simulink model "stellaris_lp_gmeter"  (R2017a)
settings: Solver=FixedStepDiscrete  StartTime=0.0  StopTime=10.0  FixedStep=0.01  RelTol=1e-3  EnableMultiTasking=on
undefined symbols (not defined in the file): C, T
libraries: stellaris_lp_lib x4
settings Model: ExtModeTrigDuration=2  Creator=peselnikmg  LastModifiedBy=Nilim
settings DataIOCC: LimitDataPoints=on  SaveFormat=Array  SignalLoggingSaveFormat=ModelDataLogs  ReturnWorkspaceOutputs=on
settings OptimizationCC: UseDivisionForNetSlopeComputation=on  UseFloatMulNetSlope=on  UseSpecifiedMinMax=on  PassReuseOutputArgsAs=Individual arguments  ExpressionDepthLimit=2147483647  ZeroExternalMemoryAtStartup=off  ZeroInternalMemoryAtStartup=off  NoFixptDivByZeroProtection=on  EfficientFloat2IntCast=on  LifeSpan=inf  MaxStackSize=64  OptimizeBlockOrder=speed
settings DebuggingCC: ReadBeforeWriteMsg=DisableAll  WriteAfterWriteMsg=DisableAll  WriteAfterReadMsg=DisableAll  MultiTaskDSMMsg=none  IntegerOverflowMsg=error  ParameterTunabilityLossMsg=error  AssertControl=DisableAll  StateNameClashWarn=warning  NonBusSignalsTreatedAsBus=error  SFInvalidInputDataAccessInChartInitDiag=error  SFTransitionOutsideNaturalParentDiag=error  SFUnreachableExecutionPathDiag=error  SFUndirectedBroadcastEventsDiag=error  SFExecutionAtInitializationDiag=none  IntegerSaturationMsg=error
settings HardwareCC: ProdBitPerPointer=32  ProdBitPerSizeT=32  ProdBitPerPtrDiffT=32  ProdLargestAtomicInteger=Long  ProdLargestAtomicFloat=Double  ProdWordSize=32  ProdHWDeviceType=ARM Compatible->ARM Cortex
settings ModelReferenceCC: UpdateModelReferenceTargets=IfOutOfDate  PropagateSignalLabelsOutOfModel=off
settings SFSimCC: SFSimEcho=off  MATLABDynamicMemAlloc=off
settings RTWCC: SystemTargetFile=ert.tlc  HardwareBoard=Tiva TM4C123G Launchpad  TLCOptions=-aInlineSetEventsForThisBaseRateFcn=TLC_FALSE -aSuppressMultiTaskScheduler=TLC_FALSE -aRateBasedStepFcn=1  TemplateMakefile=ert_default_tmf  Description=Embedded Coder  GenerateReport=on  RTWVerbose=off  Toolchain=Texas Instruments Code Composer Studio v6 (Tiva)  BuildConfiguration=Faster Runs  IncludeHyperlinkInReport=on  LaunchReport=on  GenerateTraceInfo=on  GenerateTraceReport=on  GenerateTraceReportSl=on  GenerateTraceReportSf=on  GenerateTraceReportEml=on
settings CodeAppCC: ForceParamTrailComments=on  IgnoreCustomStorageClasses=off  OperatorAnnotations=on  SimulinkDataObjDesc=on  SFDataObjDesc=on  MATLABFcnDesc=on  CustomSymbolStrType=$N$R$M  InsertBlockDesc=on  MATLABSourceComments=on  EnableCustomComments=on  ReqsInCode=on
settings ERTTargetCC: UtilityFuncGeneration=Shared location  CombineSignalStateStructs=on  SuppressErrorStatus=on  SupportNonFinite=off  ParenthesesLevel=Maximum  CastingMode=Standards  EnableSignedLeftShifts=off  EnableSignedRightShifts=off
settings ConfigComp: CovMetricSettings=dw  CovHtmlReporting=on  CovSaveCumulativeToWorkspaceVar=on  CovSaveSingleToWorkspaceVar=on  CovExternalEMLEnable=off

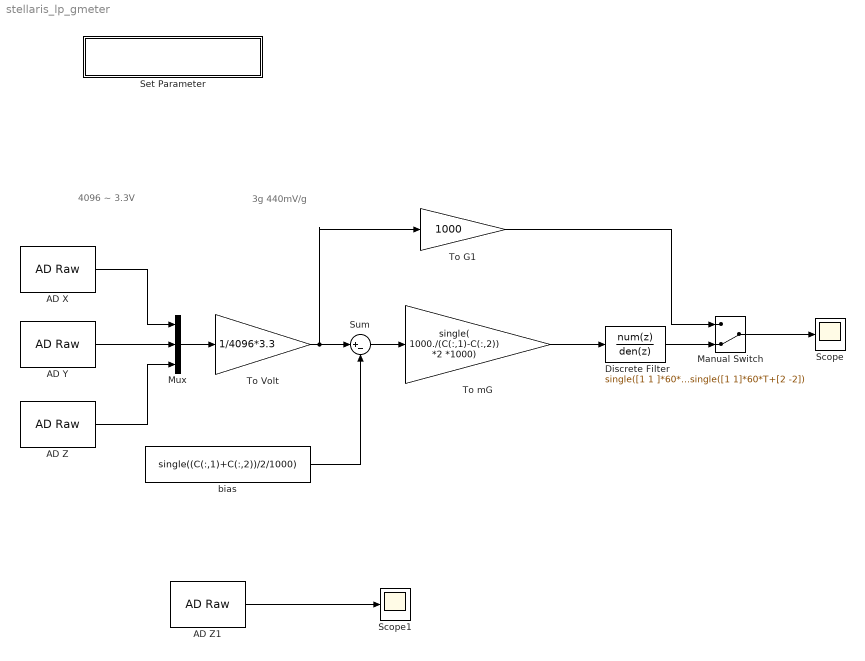
== system stellaris_lp_gmeter ==
  note: 4096 ~ 3.3V
  note: 3g 440mV/g
  AD X : stellaris_lp_lib/ADC/AD Raw  ch="1   PE3"  sample_time=0.01
      settings: SourceProductName=Run on Stellaris LaunchPad
  AD Y : stellaris_lp_lib/ADC/AD Raw  ch="2   PE2"  sample_time=0.01
      settings: SourceProductName=Run on Stellaris LaunchPad
  AD Z : stellaris_lp_lib/ADC/AD Raw  ch="3   PE1"  sample_time=0.01
      settings: SourceProductName=Run on Stellaris LaunchPad
  AD Z1 : stellaris_lp_lib/ADC/AD Raw  ch="4   PE0"  sample_time=0.02
      settings: SourceProductName=Run on Stellaris LaunchPad
  Discrete Filter : DiscreteFilter  Numerator=single([1 1 ]*60*T)  Denominator=single([1 1]*60*T+[2 -2])  InitialStates=single([0;0;0])
  Manual Switch : ManualSwitch  CurrentSetting=0
  Mux : Mux  Inputs=3
  Scope : Scope
  Scope1 : Scope
  Set Parameter : Subsystem
      settings: OpenFcn=|
      | C = [2375 725;2500 910;2180 625];
      | T=0.01;
      mask Display: fprintf('Double-click to set parameter')
  Sum : Sum  Inputs=|+-
  To G1 : Gain  Gain=1000  ParamDataTypeStr=single  OutDataTypeStr=single
  To Volt : Gain  Gain=1/4096*3.3  ParamDataTypeStr=single
  To mG : Gain  Gain="single(   1000./(C(:,1)-C(:,2))   *2 *1000)"  ParamDataTypeStr=single  OutDataTypeStr=single
  bias : Constant  Value=single((C(:,1)+C(:,2))/2/1000)
  wires:
  Mux/1 -> To Volt/1
  To Volt/1 -> To G1/1, Sum/1
  bias/1 -> Sum/2
  Sum/1 -> To mG/1
  AD X/1 -> Mux/1
  AD Y/1 -> Mux/2
  AD Z/1 -> Mux/3
  Manual Switch/1 -> Scope/1
  To mG/1 -> Discrete Filter/1
  To G1/1 -> Manual Switch/1
  Discrete Filter/1 -> Manual Switch/2
  AD Z1/1 -> Scope1/1

== system stellaris_lp_gmeter/Set Parameter ==
